simulink model "butterfly_simulink"  (R2020a)
settings: Solver=ode45  StartTime=0.0  StopTime=2*pi  FixedStep=0.001  MaxStep=0.01  RelTol=1e-6  AbsTol=1e-6
values from neighbouring files (symbols this model uses):
  bf = ButterflyFrame    [runButterflyFrame.m]
libraries: simulink x4
settings Model: Creator=g-oft  LastModifiedBy=g-oft

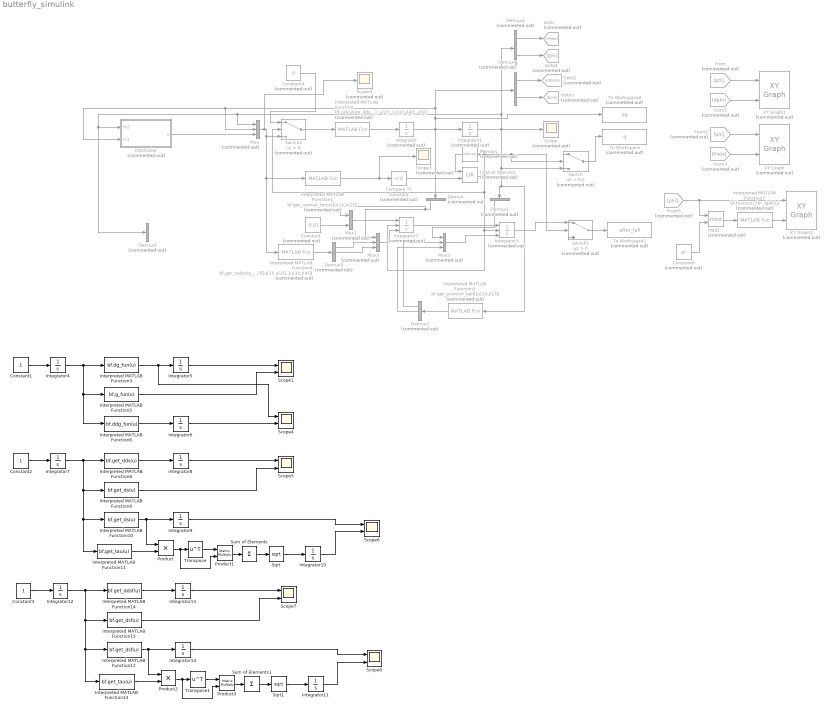
== system butterfly_simulink ==
  COntroller : Subsystem  Commented=on
  Compare To Constant : simulink/Logic and Bit Operations/Compare To Constant  Commented=on  relop=<  const=0  OutDataTypeStr=boolean
  Constant : Constant  Commented=on  Value=-9.81
  Constant1 : Constant
  Constant2 : Constant
  Constant3 : Constant
  Constant4 : Constant  Commented=on  Value=0
  Constant6 : Constant  Commented=on  Value=pi
  Demux{,1,4..5,7} (5 alike) : Demux  Commented=on  Outputs=2
  Demux2 : Demux  Commented=on  Outputs=3
  Demux3 : Demux  Commented=on  Outputs=3
  From : From  Commented=on  GotoTag=phi
  From1 : From  Commented=on  GotoTag=dphi
  From2 : From  Commented=on  GotoTag=phi
  From3 : From  Commented=on  GotoTag=theta
  From5 : From  Commented=on  GotoTag=phi
  Goto : Goto  Commented=on  GotoTag=theta
  Goto1 : Goto  Commented=on  GotoTag=phi
  Goto2 : Goto  Commented=on  GotoTag=dtheta
  Goto3 : Goto  Commented=on  GotoTag=dphi
  Integrator : Integrator  Commented=on  InitialCondition=[bf.get_dtheta(0)*bf.function_for_dphi(0);bf.function_for_dphi(0)]
  Integrator1 : Integrator  Commented=on  InitialCondition=[0;0]
  Integrator{4,7,9..12,14} (7 alike) : Integrator
  Integrator13 : Integrator  InitialCondition=bf.get_dsf(0)
  Integrator2 : Integrator  Commented=on  ExternalReset=rising  InitialConditionSource=external
  Integrator3 : Integrator  Commented=on  ExternalReset=rising  InitialConditionSource=external
  Integrator5 : Integrator  InitialCondition=bf.g_fun(0)
  Integrator6 : Integrator  InitialCondition=bf.dg_fun(0)
  Integrator8 : Integrator  InitialCondition=bf.get_ds(0)
  Interpreted MATLAB Function : MATLABFcn  Commented=on  MATLABFcn=bf.calculate_ddq([u(1); u(2)], [u(3);u(4)], u(5))
  Interpreted MATLAB Function1 : MATLABFcn  Commented=on  MATLABFcn=bf.get_normal_force([u(1); u(2)])
  Interpreted MATLAB Function10 : MATLABFcn  MATLABFcn=bf.get_ds(u)
  Interpreted MATLAB Function11 : MATLABFcn  MATLABFcn=bf.get_tau(u)
  Interpreted MATLAB Function12 : MATLABFcn  MATLABFcn=bf.get_dsf(u)
  Interpreted MATLAB Function13 : MATLABFcn  MATLABFcn=bf.get_tau(u)
  Interpreted MATLAB Function14 : MATLABFcn  MATLABFcn=bf.get_ddsf(u)
  Interpreted MATLAB Function15 : MATLABFcn  MATLABFcn=bf.get_dsf(u)
  Interpreted MATLAB Function2 : MATLABFcn  Commented=on  MATLABFcn=bf.get_position_ball([u(1);u(2)])
  Interpreted MATLAB Function3 : MATLABFcn  MATLABFcn=bf.dg_fun(u)
  Interpreted MATLAB Function4 : MATLABFcn  Commented=on  MATLABFcn=bf.get_velocity_ball([u(1); u(2)], [u(3);u(4)])
  Interpreted MATLAB Function5 : MATLABFcn  MATLABFcn=bf.g_fun(u)
  Interpreted MATLAB Function6 : MATLABFcn  MATLABFcn=bf.ddg_fun(u)
  Interpreted MATLAB Function7 : MATLABFcn  Commented=on  MATLABFcn=bf.function_for_dphi(u)
  Interpreted MATLAB Function8 : MATLABFcn  MATLABFcn=bf.get_dds(u)
  Interpreted MATLAB Function9 : MATLABFcn  MATLABFcn=bf.get_ds(u)
  Logical Operator : Logic  Commented=on  Operator=OR  AllPortsSameDT=off  OutDataTypeStr=boolean
  Memory : Memory  Commented=on
  Mod1 : Math  Commented=on  Operator=mod  SaturateOnIntegerOverflow=on
  Mux{,1..3} (4 alike) : Mux  Commented=on  Inputs=3
  Product : Product
  Product1 : Product  Multiplication=Matrix(*)
  Product2 : Product
  Product3 : Product  Multiplication=Matrix(*)
  Scope : Scope  Commented=on
  Scope{1,4..8} (6 alike) : Scope  NumInputPorts=2
  Scope2 : Scope  Commented=on
  Scope3 : Scope  Commented=on
  Sqrt : Sqrt  SaturateOnIntegerOverflow=on
  Sqrt1 : Sqrt  SaturateOnIntegerOverflow=on
  Sum of Elements : Sum  Inputs=+
  Sum of Elements1 : Sum  Inputs=+
  Switch : Switch  Commented=on  Criteria=u2 > Threshold  Threshold=0.5
  Switch1 : Switch  Commented=on  Criteria=u2 > Threshold
  Switch2 : Switch  Commented=on  Criteria=u2 > Threshold
  To Workspace : ToWorkspace  Commented=on  VariableName=q  SampleTime=-1
  To Workspace1 : ToWorkspace  Commented=on  VariableName=after_fall  SampleTime=-1
  To Workspace2 : ToWorkspace  Commented=on  VariableName=dq  SampleTime=-1
  Transpose : Math  Operator=transpose  SaturateOnIntegerOverflow=on
  Transpose1 : Math  Operator=transpose  SaturateOnIntegerOverflow=on
  XY Graph : simulink/Sinks/XY Graph  Commented=on  xmin=0  xmax=10  ymin=-1  ymax=10  st=-1
  XY Graph1 : simulink/Sinks/XY Graph  Commented=on  xmin=0  xmax=10  ymin=0  ymax=3  st=-1
  XY Graph2 : simulink/Sinks/XY Graph  Commented=on  xmin=0  xmax=10  ymin=0  ymax=3  st=-1
  wires:
  Interpreted MATLAB Function/1 -> Integrator/1
  Integrator/1 -> Demux/1, To Workspace2/1, Demux7/1, Mux/2, COntroller/2(In1), Integrator1/1
  Switch/1 -> To Workspace/1
  Mux1/1 -> Integrator2/1
  Constant/1 -> Mux1/3
  Integrator2/1 -> Integrator3/1
  Memory/1 -> Logical Operator/1
  Logical Operator/1 -> Switch2/2, Integrator2/2, Integrator3/2, Memory/1, Switch1/2, Switch/2
  Interpreted MATLAB Function1/1 -> Scope3/1, Compare To Constant/1
  Compare To Constant/1 -> Logical Operator/2
  Mux2/1 -> Integrator3/3
  Demux/1 -> Mux1/1, Mux3/1
  Mux3/1 -> Integrator2/3
  Demux1/1 -> Mux2/1
  Demux2/1 -> Mux2/2
  Demux2/2 -> Mux2/3
  Demux3/1 -> Mux3/2
  Demux3/2 -> Mux3/3
  Interpreted MATLAB Function4/1 -> Demux3/1
  Switch1/1 -> To Workspace1/1
  Interpreted MATLAB Function2/1 -> Demux2/1
  Integrator3/1 -> Switch1/1
  Mux/1 -> Scope2/1, Interpreted MATLAB Function4/1, Interpreted MATLAB Function1/1, Switch2/3
  Demux4/1 -> Goto/1
  Demux4/2 -> Goto1/1
  Demux7/2 -> Goto3/1
  Demux7/1 -> Goto2/1
  Integrator1/1 -> Scope/1, Interpreted MATLAB Function2/1, Demux1/1, Switch/3, Mux/1, Demux5/1, COntroller/1(In2), Demux4/1
  From/1 -> XY Graph1/1
  From1/1 -> XY Graph1/2
  From2/1 -> XY Graph/1
  From3/1 -> XY Graph/2
  Switch2/1 -> Interpreted MATLAB Function/1
  Constant4/1 -> Switch2/1
  From5/1 -> Mod1/1, XY Graph2/1
  Interpreted MATLAB Function7/1 -> XY Graph2/2
  Mod1/1 -> Interpreted MATLAB Function7/1
  Constant6/1 -> Mod1/2
  COntroller/1(u) -> Mux/3
  Constant1/1 -> Integrator4/1
  Integrator4/1 -> Interpreted MATLAB Function6/1, Interpreted MATLAB Function5/1, Interpreted MATLAB Function3/1
  Interpreted MATLAB Function3/1 -> Scope4/1, Integrator5/1
  Interpreted MATLAB Function5/1 -> Scope1/2
  Integrator5/1 -> Scope1/1
  Interpreted MATLAB Function6/1 -> Integrator6/1
  Integrator6/1 -> Scope4/2
  Interpreted MATLAB Function8/1 -> Integrator8/1
  Integrator7/1 -> Interpreted MATLAB Function11/1, Interpreted MATLAB Function10/1, Interpreted MATLAB Function9/1, Interpreted MATLAB Function8/1
  Constant2/1 -> Integrator7/1
  Interpreted MATLAB Function9/1 -> Scope5/2
  Integrator8/1 -> Scope5/1
  Interpreted MATLAB Function10/1 -> Product/1, Integrator9/1
  Integrator9/1 -> Scope6/1
  Product1/1 -> Sum of Elements/1
  Sum of Elements/1 -> Sqrt/1
  Sqrt/1 -> Integrator10/1
  Interpreted MATLAB Function11/1 -> Product/2
  Product/1 -> Product1/2, Transpose/1
  Transpose/1 -> Product1/1
  Integrator10/1 -> Scope6/2
  Interpreted MATLAB Function13/1 -> Product2/2
  Integrator14/1 -> Scope8/1
  Integrator13/1 -> Scope7/1
  Interpreted MATLAB Function15/1 -> Scope7/2
  Integrator12/1 -> Interpreted MATLAB Function13/1, Interpreted MATLAB Function12/1, Interpreted MATLAB Function15/1, Interpreted MATLAB Function14/1
  Constant3/1 -> Integrator12/1
  Interpreted MATLAB Function14/1 -> Integrator13/1
  Sum of Elements1/1 -> Sqrt1/1
  Integrator11/1 -> Scope8/2
  Transpose1/1 -> Product3/1
  Interpreted MATLAB Function12/1 -> Product2/1, Integrator14/1
  Product2/1 -> Product3/2, Transpose1/1
  Sqrt1/1 -> Integrator11/1
  Product3/1 -> Sum of Elements1/1

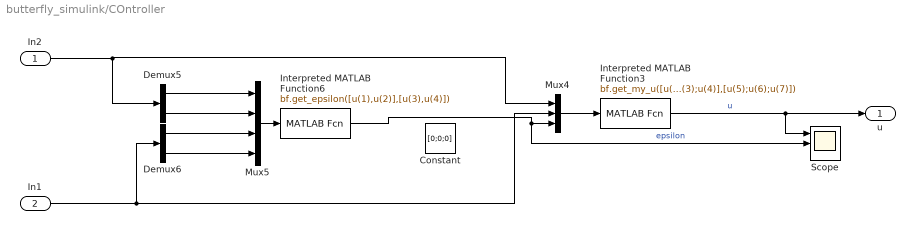
== system butterfly_simulink/COntroller ==
  In2 : Inport
  In1 : Inport  Port=2
  Constant : Constant  Value=[0;0;0]
  Demux5 : Demux  Outputs=2
  Demux6 : Demux  Outputs=2
  Interpreted MATLAB Function3 : MATLABFcn  MATLABFcn=bf.get_my_u([u(1);u(2)],[u(3);u(4)],[u(5);u(6);u(7)])
  Interpreted MATLAB Function6 : MATLABFcn  MATLABFcn=bf.get_epsilon([u(1),u(2)],[u(3),u(4)])
  Mux4 : Mux  Inputs=3
  Mux5 : Mux
  Scope : Scope  NumInputPorts=3
  u : Outport
  wires:
  Interpreted MATLAB Function3/1 -> u/1, Scope/1  "u"
  In2/1 -> Demux5/1, Mux4/1
  Mux5/1 -> Interpreted MATLAB Function6/1
  Demux5/2 -> Mux5/2
  Demux6/1 -> Mux5/3
  In1/1 -> Mux4/2, Demux6/1
  Demux5/1 -> Mux5/1
  Mux4/1 -> Interpreted MATLAB Function3/1
  Demux6/2 -> Mux5/4
  Interpreted MATLAB Function6/1 -> Scope/2, Mux4/3  "epsilon"
